simulink model "projectile"  (R2016b)
settings: Solver=FixedStepAuto  StartTime=0.0  StopTime=0.5  FixedStep=0.05  RelTol=1e-3
settings Model: Creator=jeremycrowley  LastModifiedBy=jeremycrowley

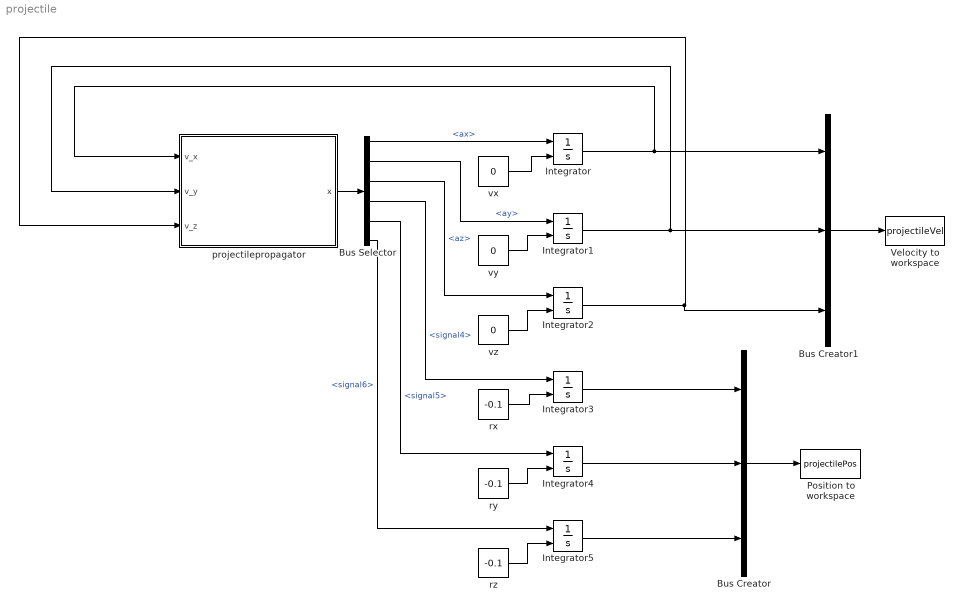
== system projectile ==
  Bus Creator : BusCreator  Inputs=3
  Bus Creator1 : BusCreator  Inputs=3
  Bus Selector : BusSelector  OutputSignals=ax,ay,az,signal4,signal5,signal6
  Integrator{,1..5} (6 alike) : Integrator  InitialConditionSource=external
  Position to workspace : ToWorkspace  VariableName=projectilePos  SampleTime=-1
  Velocity to workspace : ToWorkspace  VariableName=projectileVel  SampleTime=-1
  projectilepropagator : Subsystem
  rx : Constant  Value=-0.1
  ry : Constant  Value=-0.1
  rz : Constant  Value=-0.1
  vx : Constant  Value=0
  vy : Constant  Value=0
  vz : Constant  Value=0
  wires:
  Bus Selector/1 -> Integrator/1  "<ax>"
  Bus Selector/2 -> Integrator1/1  "<ay>"
  Bus Selector/3 -> Integrator2/1  "<az>"
  vx/1 -> Integrator/2
  vy/1 -> Integrator1/2
  vz/1 -> Integrator2/2
  projectilepropagator/1(x) -> Bus Selector/1
  rx/1 -> Integrator3/2
  ry/1 -> Integrator4/2
  rz/1 -> Integrator5/2
  Bus Selector/4 -> Integrator3/1  "<signal4>"
  Bus Selector/5 -> Integrator4/1  "<signal5>"
  Bus Selector/6 -> Integrator5/1  "<signal6>"
  Bus Creator/1 -> Position to workspace/1
  Integrator4/1 -> Bus Creator/2
  Integrator3/1 -> Bus Creator/1
  Integrator5/1 -> Bus Creator/3
  Bus Creator1/1 -> Velocity to workspace/1
  Integrator1/1 -> Bus Creator1/2, projectilepropagator/2(v_y)
  Integrator/1 -> Bus Creator1/1, projectilepropagator/1(v_x)
  Integrator2/1 -> Bus Creator1/3, projectilepropagator/3(v_z)

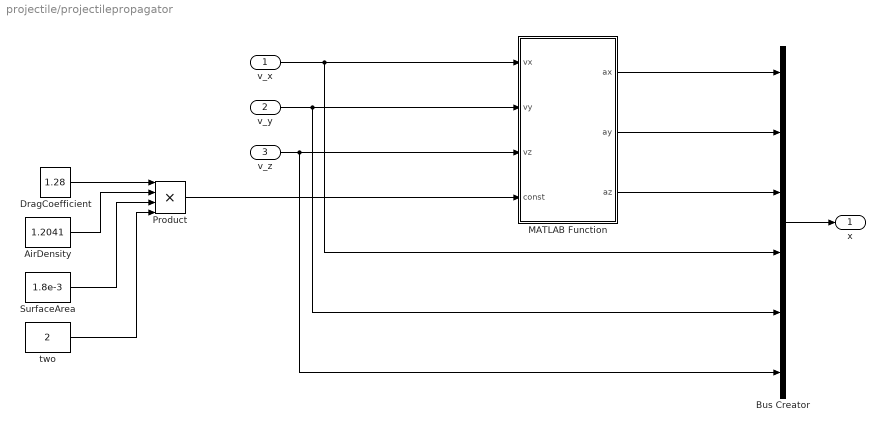
== system projectile/projectilepropagator ==
  v_x : Inport
  v_y : Inport  Port=2
  v_z : Inport  Port=3
  AirDensity : Constant  Value=1.2041
  Bus Creator : BusCreator  Inputs=6
  DragCoefficient : Constant  Value=1.28
  MATLAB Function : MATLAB Function  TreatAsAtomicUnit=on
  Product : Product  Inputs=4
  SurfaceArea : Constant  Value=1.8e-3
  two : Constant  Value=2
  x : Outport
  wires:
  DragCoefficient/1 -> Product/1
  AirDensity/1 -> Product/2
  SurfaceArea/1 -> Product/3
  v_x/1 -> MATLAB Function/1(vx), Bus Creator/4
  v_y/1 -> MATLAB Function/2(vy), Bus Creator/5
  v_z/1 -> MATLAB Function/3(vz), Bus Creator/6
  two/1 -> Product/4
  Bus Creator/1 -> x/1
  Product/1 -> MATLAB Function/4(const)
  MATLAB Function/1(ax) -> Bus Creator/1
  MATLAB Function/2(ay) -> Bus Creator/2
  MATLAB Function/3(az) -> Bus Creator/3

== matlab function projectile/projectilepropagator/MATLAB Function ==
  data: vx input; ax output; vy input; vz input; const input; ay output; az output
function [ax,ay,az] = fcn(vx, vy, vz, const)

    g = 9.81;
    
    rx = const * (vx^2);
    ry = const * (vy^2);
    rz = const * (vz^2);
    
    if(vx < 0)
        ax = rx;
    else
        ax = -rx;
    end

    if(vy < 0)
        ay = ry;
    else
        ay = -ry;
    end

    if(vz < 0)
        az = -g + rz;
    else
        az = -g - rz;
    end
    
end
